simulink model "sampleModel1658"  (R2023a)
settings: Solver=VariableStepAuto  StartTime=0.0  StopTime=10.0  RelTol=1e-3
libraries: simulink x4, hdlsllib x4
settings Model: Creator=user1  LastModifiedBy=user1

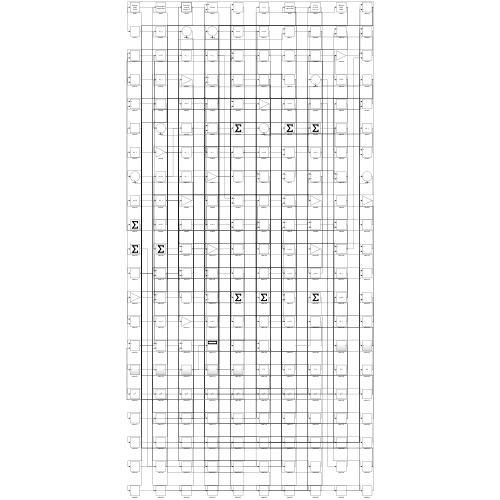
[thumbnail: Simulink's stored preview of the top-level diagram]
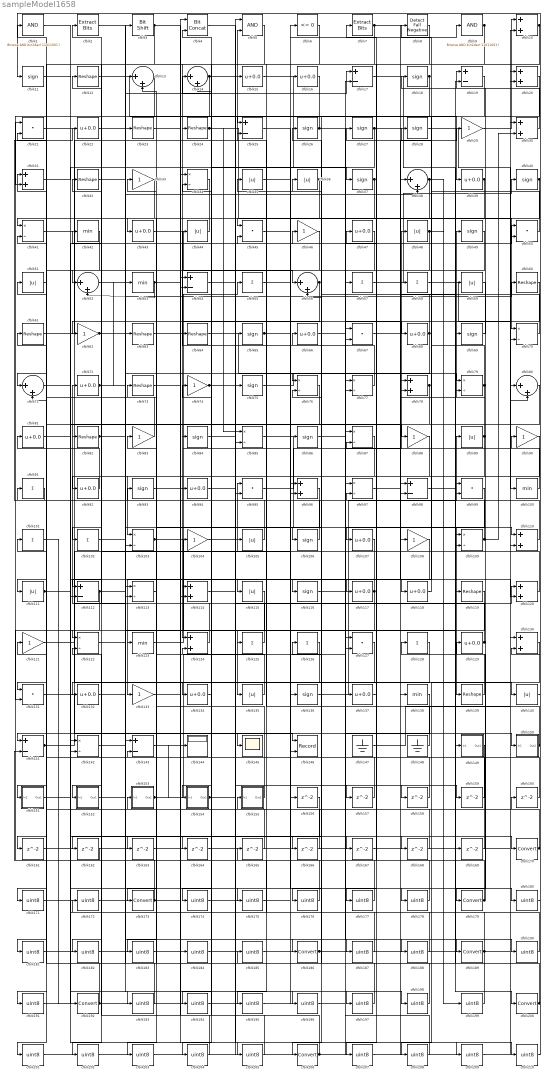
== system sampleModel1658 ==
  cfblk1 : simulink/Logic and Bit Operations/Bitwise Operator  logicop=AND  UseBitMask=on  BitMask=bin2dec('11011001')  BitMaskRealWorld=Stored Integer
      settings: LibrarySourceBlock=|
      | hdlsllib/Logic and Bit
      | Operations/Bitwise
      | Operator
  cfblk{10,20,30..31,78,96,110,114,120,124,130} (11 alike) : Sum
  cfblk{42,53,100,123,138} (5 alike) : MinMax
  cfblk{55,57..58,91,101..102,125..126,128} (9 alike) : Sum  Inputs=+
  cfblk{34,41,70,76..77,79,85,87,97,103,109,113,122,142} (14 alike) : Product  Inputs=*/  RndMeth=Zero  SaturateOnIntegerOverflow=on
  cfblk{29,33,46,62,74,83,88,90,104,108,121,133} (12 alike) : Gain
  cfblk{35..36,44,48,51,59,89,105,111,115,135,140} (12 alike) : Abs  SaturateOnIntegerOverflow=off
  cfblk{11,18,26..28,37,40,49,65,69,75,84,86,93,106,116,136} (17 alike) : Signum
  cfblk{15..16,22,39,43,47,66,68,72,81,92,94,107,117..118,129,132,134,137} (19 alike) : Bias  Bias=0.0  SaturateOnIntegerOverflow=off
  cfblk{17,19,25,54,98,112,141,143} (8 alike) : Sum  Inputs=+-
  cfblk{12,23..24,32,60..61,63..64,73,82,119,139} (12 alike) : Reshape
  cfblk{21,45,50,67,95,99,127,131} (8 alike) : DotProduct  OutDataTypeStr=Inherit: Inherit via internal rule
  cfblk{13..14,38,52,56,71,80} (7 alike) : Sum  Inputs=|++
  cfblk144 : Display
  cfblk145 : Scope
  cfblk146 : Record  FileSettingsInternal="{\"entries\":[{\"content\":{\"excelSettings\":{\"content\":{},\"type\":\"Streamout.ExcelSettings\"}},\"type\":\"Streamout.FileSettingStorage\",\"uuid\":\"\"}],\"packageUris\":[\"http:\\/\\/schema.mathworks.com\\/mf0\\/streamout_blocks\\/R2020a\"],\"version\":\"1.0\"}"  Layout=[1 1]  SignalsInternal="{\"entries\":[{\"content\":{\"signals\":[{\"content\":{\"blockPath\":[],\"dimensions\":[1],\"domain\":\"\",\"lineColor\":\"#a2142f\",\"plots\":[1],\"port\":1,\"signalID\":2602,\"signalName\":\"XY Graph:1\"},\"type\":\"RecordBlkView.Signal\",\"uuid\":\"\"},{\"content\":{\"blockPath\":[],\"dimensions\":[1],\"domain\":\"\",\"lineColor\":\"#139fff\",\"plots\":[1],\"port\":2,\"signalID\":2605,\"signalName\":\"XY Graph:2\"},\"type\":\"RecordBlkView.Signal\",\"uuid\":\"\"}]},\"type\":\"RecordBlkView.InputSignals\",\"uuid\":\"\"}],\"packageUris\":[\"http:\\/\\/schema.mathworks.com\\/mf0\\/streamout_blocks\\/R2020a\"],\"version\":\"1.0\"}"  VisualizationBindings="{\"xyplotplugin\":{\"info\":[{\"series\":[{\"bindingParametersList\":[{\"parameter\":\"X-Axis\",\"signalID\":2602,\"signalName\":\"XY Graph:1\"},{\"parameter\":\"Y-Axis\",\"signalID\":2605,\"signalName\":\"XY Graph:2\"}],\"seriesID\":11351}],\"subplotID\":1}]}}"  CompatibilityTag=XY  st=-1
  cfblk147 : Ground
  cfblk148 : Ground
  cfblk149 : Subsystem
      settings: LibrarySourceBlock=|
      | hdlsllib/Ports &
      | Subsystems/Subsystem
  cfblk150 : Subsystem
      settings: LibrarySourceBlock=|
      | hdlsllib/Ports &
      | Subsystems/Subsystem
  cfblk151 : Subsystem
      settings: LibrarySourceBlock=|
      | hdlsllib/Ports &
      | Subsystems/Subsystem
  cfblk152 : Subsystem
      settings: LibrarySourceBlock=|
      | hdlsllib/Ports &
      | Subsystems/Subsystem
  cfblk153 : Subsystem
      settings: LibrarySourceBlock=|
      | hdlsllib/Ports &
      | Subsystems/Subsystem
  cfblk154 : Subsystem
      settings: LibrarySourceBlock=|
      | hdlsllib/Ports &
      | Subsystems/Subsystem
  cfblk155 : Subsystem
      settings: LibrarySourceBlock=|
      | hdlsllib/Ports &
      | Subsystems/Subsystem
  cfblk{156..169} (14 alike) : Delay  SampleTime=1
  cfblk{170,173,179,186,189,192,200,206} (8 alike) : DataTypeConversion  SaturateOnIntegerOverflow=off  RndMeth=Floor
  cfblk{171..172,174..178,180..185,187..188,190..191,193..199,201..205,207..210} (33 alike) : DataTypeConversion  OutDataTypeStr=uint8  SaturateOnIntegerOverflow=off  RndMeth=Floor
  cfblk2 : simulink/Logic and Bit Operations/Extract Bits  bitsToExtract=Upper half  numBits=8  bitIdxRange=[0 7]  outScalingMode=Preserve fixed-point scaling
      settings: LibrarySourceBlock=|
      | hdlsllib/Logic and Bit
      | Operations/Extract Bits
  cfblk3 : hdlsllib/Logic and Bit Operations/Bit Shift  mode=Shift Left Logical  N=0
  cfblk4 : hdlsllib/Logic and Bit Operations/Bit Concat  numInputs=2
  cfblk5 : Logic  AllPortsSameDT=off  OutDataTypeStr=boolean
  cfblk6 : hdlsllib/Logic and Bit Operations/Compare To Zero  relop=<=  OutDataTypeStr=boolean
  cfblk7 : simulink/Logic and Bit Operations/Extract Bits  bitsToExtract=Upper half  numBits=8  bitIdxRange=[0 7]  outScalingMode=Preserve fixed-point scaling
      settings: LibrarySourceBlock=|
      | hdlsllib/Logic and Bit
      | Operations/Extract Bits
  cfblk8 : hdlsllib/Logic and Bit Operations/Detect Fall Negative  vinit=0  OutDataTypeStr=boolean
  cfblk9 : simulink/Logic and Bit Operations/Bitwise Operator  logicop=AND  UseBitMask=on  BitMask=bin2dec('11011001')  BitMaskRealWorld=Stored Integer
      settings: LibrarySourceBlock=|
      | hdlsllib/Logic and Bit
      | Operations/Bitwise
      | Operator
  wires:
  cfblk89/1 -> cfblk49/1, cfblk107/1
  cfblk21/1 -> cfblk140/1
  cfblk59/1 -> cfblk103/1
  cfblk43/1 -> cfblk56/1
  cfblk69/1 -> cfblk19/1
  cfblk129/1 -> cfblk72/1, cfblk25/2
  cfblk123/1 -> cfblk55/1
  cfblk91/1 -> cfblk22/1
  cfblk122/1 -> cfblk23/1
  cfblk12/1 -> cfblk39/1
  cfblk17/1 -> cfblk69/1
  cfblk96/1 -> cfblk173/1
  cfblk98/1 -> cfblk200/1
  cfblk41/1 -> cfblk3/1
  cfblk155/1(Out1) -> cfblk83/1
  cfblk13/1 -> cfblk102/1
  cfblk37/1 -> cfblk106/1, cfblk154/1(In1)
  cfblk10/1 -> cfblk124/1, cfblk62/1, cfblk85/2
  cfblk56/1 -> cfblk122/1, cfblk182/1
  cfblk85/1 -> cfblk139/1
  cfblk118/1 -> cfblk28/1
  cfblk134/1 -> cfblk74/1
  cfblk135/1 -> cfblk93/1
  cfblk104/1 -> cfblk95/1
  cfblk105/1 -> cfblk73/1
  cfblk82/1 -> cfblk110/1, cfblk60/1, cfblk167/1
  cfblk139/1 -> cfblk128/1
  cfblk117/1 -> cfblk115/1, cfblk191/1
  cfblk35/1 -> cfblk136/1
  cfblk119/1 -> cfblk135/1
  cfblk75/1 -> cfblk79/1
  cfblk103/1 -> cfblk149/1(In1), cfblk117/1
  cfblk78/1 -> cfblk141/1, cfblk204/1
  cfblk109/1 -> cfblk82/1, cfblk30/2
  cfblk61/1 -> cfblk5/2
  cfblk64/1 -> cfblk76/1
  cfblk148/1 -> cfblk126/1
  cfblk29/1 -> cfblk10/1
  cfblk77/1 -> cfblk44/1
  cfblk38/1 -> cfblk41/1, cfblk199/1
  cfblk153/1(Out1) -> cfblk67/1, cfblk144/1
  cfblk154/1(Out1) -> cfblk65/1, cfblk120/1
  cfblk152/1(Out1) -> cfblk63/1
  cfblk30/1 -> cfblk18/1
  cfblk57/1 -> cfblk40/1
  cfblk121/1 -> cfblk86/1
  cfblk100/1 -> cfblk47/1
  cfblk53/1 -> cfblk52/2, cfblk187/1
  cfblk107/1 -> cfblk133/1
  cfblk33/1 -> cfblk131/1
  cfblk74/1 -> cfblk75/1, cfblk210/1
  cfblk120/1 -> cfblk32/1
  cfblk95/1 -> cfblk48/1
  cfblk36/1 -> cfblk45/1, cfblk92/1
  cfblk132/1 -> cfblk134/1
  cfblk81/1 -> cfblk45/2
  cfblk88/1 -> cfblk112/1
  cfblk113/1 -> cfblk33/1
  cfblk4/1 -> cfblk186/1
  cfblk24/1 -> cfblk70/1, cfblk85/1
  cfblk19/1 -> cfblk118/1
  cfblk106/1 -> cfblk21/2
  cfblk136/1 -> cfblk89/1
  cfblk28/1 -> cfblk70/2
  cfblk70/1 -> cfblk36/1
  cfblk140/1 -> cfblk11/1
  cfblk92/1 -> cfblk31/1
  cfblk46/1 -> cfblk114/1
  cfblk142/1 -> cfblk189/1
  cfblk14/1 -> cfblk146/2, cfblk201/1
  cfblk101/1 -> cfblk192/1
  cfblk125/1 -> cfblk2/1
  cfblk72/1 -> cfblk104/1, cfblk53/1
  cfblk97/1 -> cfblk29/1
  cfblk124/1 -> cfblk12/1
  cfblk131/1 -> cfblk146/1
  cfblk141/1 -> cfblk13/1, cfblk50/2
  cfblk3/1 -> cfblk71/1, cfblk109/1
  cfblk48/1 -> cfblk116/1, cfblk169/1
  cfblk32/1 -> cfblk125/1
  cfblk62/1 -> cfblk152/1(In1), cfblk88/1, cfblk198/1
  cfblk90/1 -> cfblk179/1
  cfblk63/1 -> cfblk68/1
  cfblk18/1 -> cfblk114/2, cfblk31/2
  cfblk7/1 -> cfblk14/2, cfblk52/1, cfblk79/2
  cfblk11/1 -> cfblk84/1
  cfblk60/1 -> cfblk67/2
  cfblk137/1 -> cfblk7/1
  cfblk79/1 -> cfblk8/1, cfblk78/2
  cfblk50/1 -> cfblk27/1
  cfblk39/1 -> cfblk132/1, cfblk99/2
  cfblk52/1 -> cfblk113/1
  cfblk58/1 -> cfblk100/1
  cfblk108/1 -> cfblk206/1
  cfblk15/1 -> cfblk77/2
  cfblk44/1 -> cfblk43/1
  cfblk31/1 -> cfblk37/1
  cfblk126/1 -> cfblk145/1
  cfblk68/1 -> cfblk35/1, cfblk103/2
  cfblk67/1 -> cfblk59/1
  cfblk86/1 -> cfblk137/1
  cfblk83/1 -> cfblk51/1
  cfblk66/1 -> cfblk150/1(In1)
  cfblk9/1 -> cfblk94/1, cfblk195/1
  cfblk42/1 -> cfblk111/1
  cfblk110/1 -> cfblk42/1
  cfblk54/1 -> cfblk170/1
  cfblk22/1 -> cfblk113/2
  cfblk102/1 -> cfblk50/1
  cfblk76/1 -> cfblk112/2
  cfblk26/1 -> cfblk25/1, cfblk158/1
  cfblk149/1(Out1) -> cfblk155/1(In1)
  cfblk65/1 -> cfblk9/1, cfblk178/1
  cfblk27/1 -> cfblk64/1, cfblk120/2
  cfblk150/1(Out1) -> cfblk97/2, cfblk105/1
  cfblk16/1 -> cfblk24/1
  cfblk111/1 -> cfblk119/1, cfblk175/1, cfblk205/1
  cfblk94/1 -> cfblk46/1
  cfblk112/1 -> cfblk38/2, cfblk131/2, cfblk17/1
  cfblk49/1 -> cfblk95/2
  cfblk93/1 -> cfblk6/1
  cfblk114/1 -> cfblk58/1
  cfblk40/1 -> cfblk123/1, cfblk56/2
  cfblk147/1 -> cfblk30/1
  cfblk51/1 -> cfblk151/1(In1)
  cfblk45/1 -> cfblk156/1
  cfblk84/1 -> cfblk157/1
  cfblk157/1 -> cfblk14/1
  cfblk158/1 -> cfblk13/2
  cfblk25/1 -> cfblk159/1
  cfblk159/1 -> cfblk71/2
  cfblk160/1 -> cfblk76/2
  cfblk47/1 -> cfblk161/1
  cfblk161/1 -> cfblk78/1
  cfblk128/1 -> cfblk162/1
  cfblk162/1 -> cfblk141/2
  cfblk151/1(Out1) -> cfblk163/1
  cfblk163/1 -> cfblk10/2
  cfblk115/1 -> cfblk164/1
  cfblk164/1 -> cfblk38/1
  cfblk165/1 -> cfblk124/2
  cfblk20/1 -> cfblk166/1
  cfblk166/1 -> cfblk41/2
  cfblk167/1 -> cfblk109/2
  cfblk55/1 -> cfblk168/1
  cfblk168/1 -> cfblk97/1
  cfblk169/1 -> cfblk1/1
  cfblk170/1 -> cfblk160/1, cfblk26/1
  cfblk5/1 -> cfblk171/1
  cfblk171/1 -> cfblk54/1
  cfblk172/1 -> cfblk54/2
  cfblk173/1 -> cfblk153/1(In1), cfblk21/1
  cfblk6/1 -> cfblk174/1
  cfblk174/1 -> cfblk96/1
  cfblk175/1 -> cfblk96/2
  cfblk87/1 -> cfblk176/1
  cfblk176/1 -> cfblk91/1
  cfblk8/1 -> cfblk177/1
  cfblk177/1 -> cfblk87/1
  cfblk178/1 -> cfblk87/2
  cfblk179/1 -> cfblk129/1, cfblk121/1
  cfblk1/1 -> cfblk180/1
  cfblk180/1 -> cfblk90/1
  cfblk138/1 -> cfblk181/1
  cfblk181/1 -> cfblk20/1
  cfblk182/1 -> cfblk138/1
  cfblk80/1 -> cfblk183/1
  cfblk183/1 -> cfblk19/2
  cfblk23/1 -> cfblk184/1
  cfblk184/1 -> cfblk80/1
  cfblk185/1 -> cfblk80/2
  cfblk186/1 -> cfblk17/2, cfblk20/2
  cfblk187/1 -> cfblk4/1
  cfblk133/1 -> cfblk188/1
  cfblk188/1 -> cfblk4/2
  cfblk189/1 -> cfblk185/1, cfblk172/1, cfblk165/1
  cfblk116/1 -> cfblk190/1
  cfblk190/1 -> cfblk142/1
  cfblk191/1 -> cfblk142/2
  cfblk192/1 -> cfblk16/1, cfblk81/1
  cfblk71/1 -> cfblk193/1
  cfblk193/1 -> cfblk101/1
  cfblk127/1 -> cfblk194/1
  cfblk194/1 -> cfblk5/1
  cfblk195/1 -> cfblk127/1
  cfblk2/1 -> cfblk196/1
  cfblk196/1 -> cfblk127/2
  cfblk143/1 -> cfblk197/1
  cfblk197/1 -> cfblk61/1
  cfblk198/1 -> cfblk143/1
  cfblk199/1 -> cfblk143/2
  cfblk200/1 -> cfblk99/1, cfblk66/1
  cfblk201/1 -> cfblk98/1
  cfblk156/1 -> cfblk202/1
  cfblk202/1 -> cfblk98/2
  cfblk34/1 -> cfblk203/1
  cfblk203/1 -> cfblk15/1
  cfblk204/1 -> cfblk34/1
  cfblk205/1 -> cfblk34/2
  cfblk206/1 -> cfblk57/1, cfblk122/2, cfblk110/2
  cfblk99/1 -> cfblk207/1
  cfblk207/1 -> cfblk108/1
  cfblk130/1 -> cfblk208/1
  cfblk208/1 -> cfblk77/1
  cfblk73/1 -> cfblk209/1
  cfblk209/1 -> cfblk130/1
  cfblk210/1 -> cfblk130/2

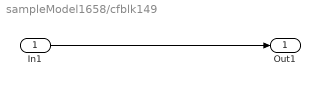
== system sampleModel1658/cfblk149 ==
  In1 : Inport
  Out1 : Outport
  wires:
  In1/1 -> Out1/1

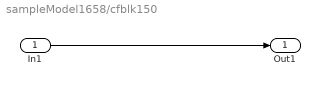
== system sampleModel1658/cfblk150 ==
  In1 : Inport
  Out1 : Outport
  wires:
  In1/1 -> Out1/1

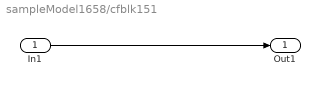
== system sampleModel1658/cfblk151 ==
  In1 : Inport
  Out1 : Outport
  wires:
  In1/1 -> Out1/1

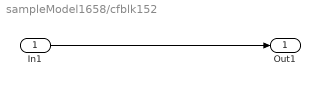
== system sampleModel1658/cfblk152 ==
  In1 : Inport
  Out1 : Outport
  wires:
  In1/1 -> Out1/1

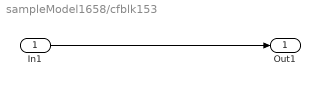
== system sampleModel1658/cfblk153 ==
  In1 : Inport
  Out1 : Outport
  wires:
  In1/1 -> Out1/1

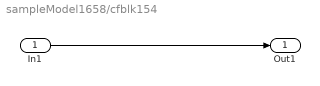
== system sampleModel1658/cfblk154 ==
  In1 : Inport
  Out1 : Outport
  wires:
  In1/1 -> Out1/1

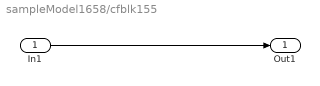
== system sampleModel1658/cfblk155 ==
  In1 : Inport
  Out1 : Outport
  wires:
  In1/1 -> Out1/1
